simulink model "untitled1"  (R2023b)
settings: Solver=VariableStepAuto  StartTime=0.0  StopTime=10.0  RelTol=1e-3
values from neighbouring files (symbols this model uses):
  A = [0        0       -k2/m2     k2/m2      0 ... (first row only)    [anews.m]
  A1 = [-cs/m2   cs/m2      -k2/m2     k2/m2      0 ... (first row only)    [anews.m]
  B = [-1/m2 ... (first row only)    [anews.m]
  B1 = [0 ... (first row only)    [anews.m]
  C = [-k2/m2     k2/m2     0      0     0 ... (first row only)    [anews.m]
  C1 = [-k2/m2     k2/m2    -cs/m2   cs/m2     0 ... (first row only)    [anews.m]
  D = [-1/m2 ... (first row only)    [anews.m]
  D1 = [0 ... (first row only)    [anews.m]
undefined symbols (not defined in the file or in its folder): Kc
libraries: simulink x1
settings Model: Creator=LENOVO  LastModifiedBy=12513
settings SolverCC: AlgebraicLoopSolver=TrustRegion
settings DataIOCC: ReturnWorkspaceOutputs=off
settings DebuggingCC: UnconnectedInputMsg=warning  UnconnectedOutputMsg=warning  UnconnectedLineMsg=warning  ArithmeticOperatorsInVariantConditions=warning
settings ModelReferenceCC: EnableRefExpFcnMdlSchedulingChecks=on
settings SFSimCC: SimUseLocalCustomCode=off  CustomCodeUndefinedFunction=UseInterfaceOnly
settings RTWCC: RTWUseLocalCustomCode=off

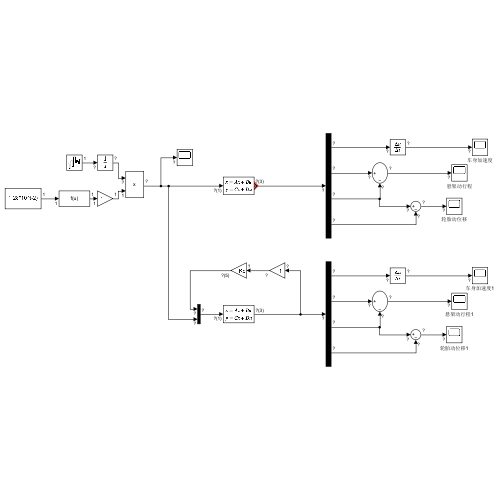
[thumbnail: Simulink's stored preview of the top-level diagram]
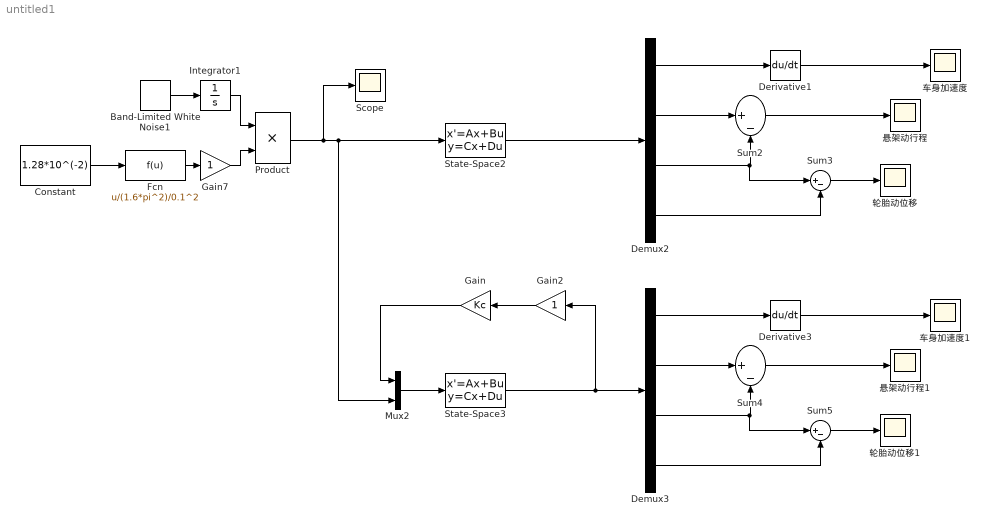
== system untitled1 ==
  Band-Limited White Noise1 : simulink/Sources/Band-Limited White Noise  Cov=[0.1]  Ts=0.1  seed=[23341]
  Constant : Constant  Value=1.28*10^(-2)
  Demux2 : Demux
  Demux3 : Demux
  Derivative1 : Derivative
  Derivative3 : Derivative
  Fcn : Fcn  Expr=u/(1.6*pi^2)/0.1^2
  Gain : Gain  Gain=Kc
  Gain2 : Gain
  Gain7 : Gain
  Integrator1 : Integrator
  Mux2 : Mux  Inputs=2
  Product : Product
  Scope : Scope
  State-Space2 : StateSpace  A=A1  B=B1  C=C1  D=D1  InitialCondition=0
  State-Space3 : StateSpace  A=A  B=B  C=C  D=D  InitialCondition=0
  Sum{2..5} (4 alike) : Sum  Inputs=|+-
  悬架动行程 : Scope
  悬架动行程1 : Scope
  车身加速度 : Scope
  车身加速度1 : Scope
  轮胎动位移 : Scope
  轮胎动位移1 : Scope
  wires:
  Gain7/1 -> Product/2
  Fcn/1 -> Gain7/1
  Constant/1 -> Fcn/1
  Band-Limited White Noise1/1 -> Integrator1/1
  Product/1 -> Scope/1, State-Space2/1, Mux2/2
  Integrator1/1 -> Product/1
  State-Space2/1 -> Demux2/1
  Demux2/1 -> Derivative1/1
  Derivative1/1 -> 车身加速度/1
  Demux2/2 -> Sum2/1
  Sum2/1 -> 悬架动行程/1
  Demux2/3 -> Sum3/1, Sum2/2
  Demux2/4 -> Sum3/2
  Sum3/1 -> 轮胎动位移/1
  Demux3/4 -> Sum5/2
  State-Space3/1 -> Gain2/1, Demux3/1
  Derivative3/1 -> 车身加速度1/1
  Demux3/1 -> Derivative3/1
  Demux3/3 -> Sum5/1, Sum4/2
  Demux3/2 -> Sum4/1
  Sum4/1 -> 悬架动行程1/1
  Sum5/1 -> 轮胎动位移1/1
  Mux2/1 -> State-Space3/1
  Gain2/1 -> Gain/1
  Gain/1 -> Mux2/1
